simulink model "Testing_&_Comparing"  (R2025b)
settings: Solver=VariableStepAuto  StartTime=0.0  StopTime=10.0  RelTol=1e-3
model workspace (MAT data in the model file):
  J = 5e-05
  K = 0.2
  L = 0.001
  R = 4
  Ts = 0.01
  V = 7.4
  b = 0.0005
  ki = 7.33
  kp = 9.39
libraries: SignalEditorBlockLib x1

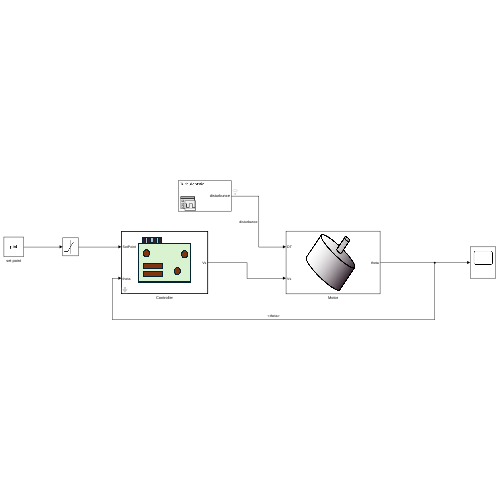
[thumbnail: Simulink's stored preview of the top-level diagram]
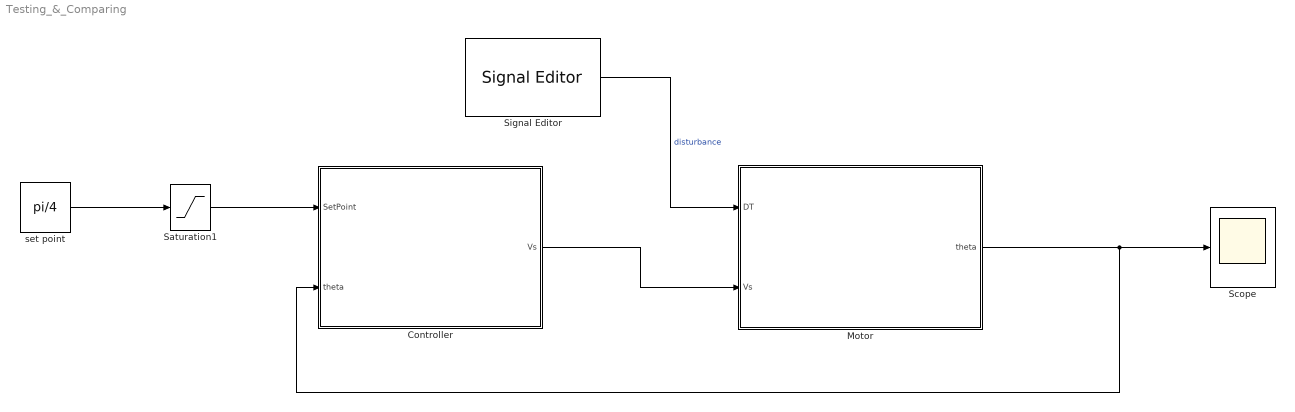
== system Testing_&_Comparing ==
  Controller : Subsystem  TreatAsAtomicUnit=on  mask{kp=9.39, ki=7.33, Ts=0.01}
      mask prompts: kp "Proportional Gain"; ki "Integral Gain"; Ts "Sample Time"
      mask Display: image('ControllerIcon.png');
  Motor : Subsystem
      mask Display: image('MotorIcon.png');
  Saturation1 : Saturate  UpperLimit=pi/4  LowerLimit=-pi/4
  Scope : Scope
      settings: ActiveDisplayYMinimum=-0.14719906446999964  ActiveDisplayYMaximum=1.063256700772913
  Signal Editor : SignalEditorBlockLib/Signal Editor  FileName=disturbance.mat  ActiveScenario=TurbulentAir  ActiveSignal=disturbunce  IsBus=off  OutputBusObjectStr=Bus: BusObject  SampleTime=0  ZeroCross=off  OutputAfterFinalValue=Setting to zero  Unit=inherit  PreserveSignalName=on  ApplySigPropsToAllScenarios=on  ApplySigPropsToAllSignals=off  SignalPropertySource=Dialog parameters
  set point : Constant  Value=pi/4
  wires:
  set point/1 -> Saturation1/1
  Motor/1(theta) -> Controller/2(theta), Scope/1
  Saturation1/1 -> Controller/1(SetPoint)
  Controller/1(Vs) -> Motor/2(Vs)
  Signal Editor/1 -> Motor/1(DT)  "disturbance"

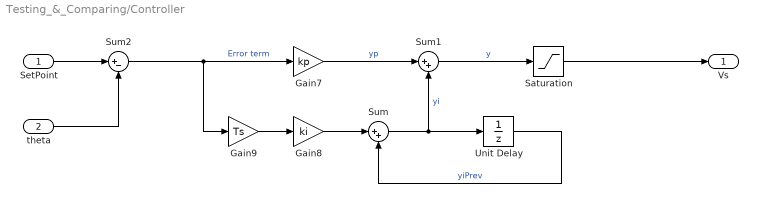
== system Testing_&_Comparing/Controller ==
  SetPoint : Inport
  theta : Inport  Port=2
  Gain7 : Gain  Gain=kp
  Gain8 : Gain  Gain=ki
  Gain9 : Gain  Gain=Ts
  Saturation : Saturate  UpperLimit=V  LowerLimit=-V
  Sum : Sum  Inputs=|++
  Sum1 : Sum  Inputs=|++
  Sum2 : Sum  Inputs=|+-
  Unit Delay : UnitDelay  InitialCondition=1  SampleTime=Ts  HasFrameUpgradeWarning=on
  Vs : Outport
  wires:
  Unit Delay/1 -> Sum/2  "yiPrev"
  Gain9/1 -> Gain8/1
  Saturation/1 -> Vs/1
  Gain8/1 -> Sum/1
  Sum2/1 -> Gain9/1, Gain7/1  "Error term"
  Sum1/1 -> Saturation/1  "y"
  SetPoint/1 -> Sum2/1
  Gain7/1 -> Sum1/1  "yp"
  Sum/1 -> Unit Delay/1, Sum1/2  "yi"
  theta/1 -> Sum2/2

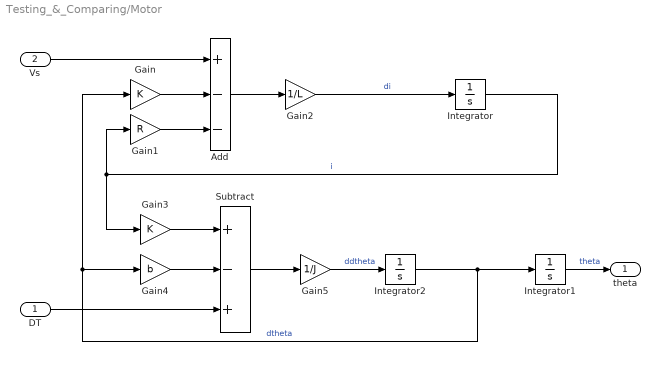
== system Testing_&_Comparing/Motor ==
  DT : Inport
  Vs : Inport  Port=2
  Add : Sum  Inputs=+--
  Gain : Gain  Gain=K
  Gain1 : Gain  Gain=R
  Gain2 : Gain  Gain=1/L
  Gain3 : Gain  Gain=K
  Gain4 : Gain  Gain=b
  Gain5 : Gain  Gain=1/J
  Integrator : Integrator
  Integrator1 : Integrator
  Integrator2 : Integrator
  Subtract : Sum  Inputs=+-+
  theta : Outport
  wires:
  Gain2/1 -> Integrator/1  "di"
  Add/1 -> Gain2/1
  Gain3/1 -> Subtract/1
  Gain1/1 -> Add/3
  Integrator/1 -> Gain1/1, Gain3/1  "i"
  Gain/1 -> Add/2
  Gain4/1 -> Subtract/2
  Integrator2/1 -> Gain/1, Gain4/1, Integrator1/1  "dtheta"
  Vs/1 -> Add/1
  Gain5/1 -> Integrator2/1  "ddtheta"
  Subtract/1 -> Gain5/1
  Integrator1/1 -> theta/1  "theta"
  DT/1 -> Subtract/3
